simulink model "bh_smd_MAIN_HELLO_ORIG"  (R2018b)
settings: Solver=ode45  StartTime=0.0  StopTime=10.0  RelTol=1e-7
undefined symbols (not defined in the file or in its folder): c, k, m, x_init, xdot_init
settings Model: Creator=bhorton  LastModifiedBy=student
settings DebuggingCC: LibraryContextMissingDiagnostic=none
settings SFSimCC: SimUseLocalCustomCode=off
settings RTWCC: RTWUseLocalCustomCode=off
settings CodeAppCC: StateflowObjectComments=on

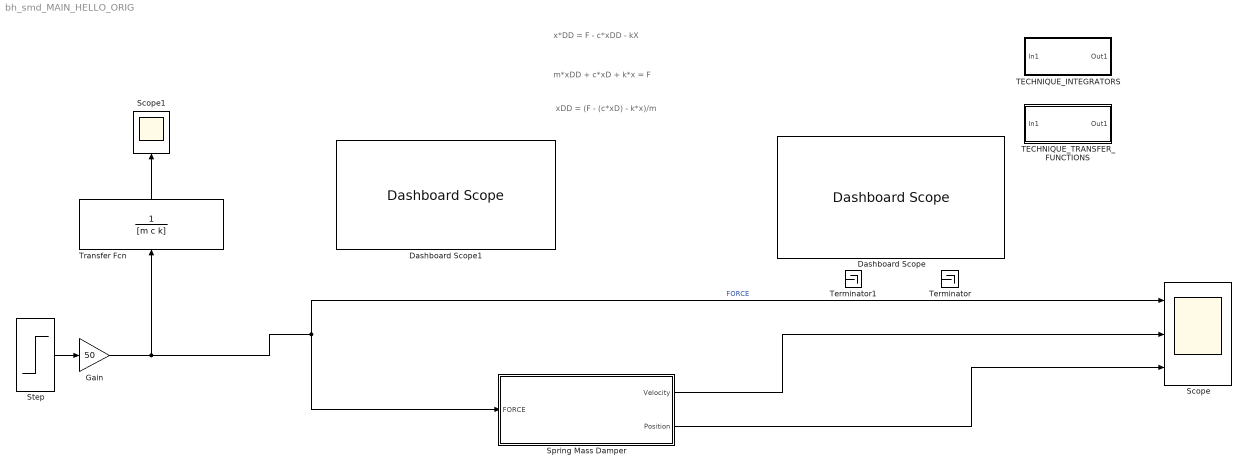
== system bh_smd_MAIN_HELLO_ORIG ==
  note: x*DD = F - c*xDD - kX
  note: xDD = (F - (c*xD) - k*x)/m
  note: m*xDD + c*xD + k*x = F
  Dashboard Scope : DashboardScope  WebBlockId=96
  Dashboard Scope1 : DashboardScope  WebBlockId=97
  Gain : Gain  Gain=50
  Scope : Scope  NumInputPorts=3
  Scope1 : Scope
  Spring Mass Damper : Subsystem
  Step : Step  Time=5  SampleTime=0
  TECHNIQUE_INTEGRATORS : Subsystem
  TECHNIQUE_TRANSFER_FUNCTIONS : Subsystem
  Terminator : Terminator
  Terminator1 : Terminator
  Transfer Fcn : TransferFcn  Denominator=[m c k]
  wires:
  Step/1 -> Gain/1
  Gain/1 -> Spring Mass Damper/1(FORCE), Scope/1, Transfer Fcn/1  "FORCE"
  Spring Mass Damper/1(Velocity) -> Scope/2
  Spring Mass Damper/2(Position) -> Scope/3
  Transfer Fcn/1 -> Scope1/1

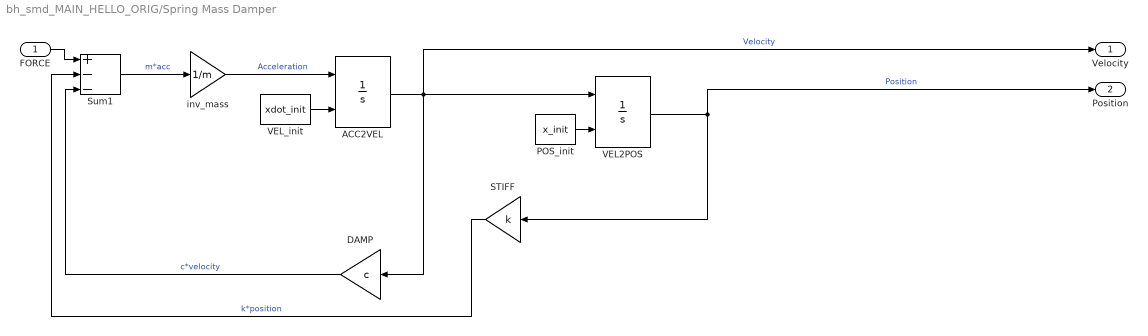
== system bh_smd_MAIN_HELLO_ORIG/Spring Mass Damper ==
  FORCE : Inport
  ACC2VEL : Integrator  InitialConditionSource=external
  "DAMP " : Gain  Gain=c
  POS_init : Constant  Value=x_init
  STIFF : Gain  Gain=k
  Sum1 : Sum  Inputs=+|-|-
  VEL2POS : Integrator  InitialConditionSource=external
  VEL_init : Constant  Value=xdot_init
  inv_mass : Gain  Gain=1/m
  Velocity : Outport
  Position : Outport  Port=2
  wires:
  Sum1/1 -> inv_mass/1  "m*acc"
  "DAMP "/1 -> Sum1/3  "c*velocity"
  VEL_init/1 -> ACC2VEL/2
  ACC2VEL/1 -> Velocity/1, "DAMP "/1, VEL2POS/1  "Velocity"
  POS_init/1 -> VEL2POS/2
  STIFF/1 -> Sum1/2  "k*position"
  inv_mass/1 -> ACC2VEL/1  "Acceleration"
  FORCE/1 -> Sum1/1
  VEL2POS/1 -> Position/1, STIFF/1  "Position"

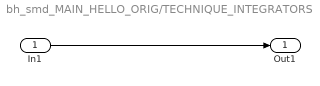
== system bh_smd_MAIN_HELLO_ORIG/TECHNIQUE_INTEGRATORS ==
  In1 : Inport
  Out1 : Outport
  wires:
  In1/1 -> Out1/1

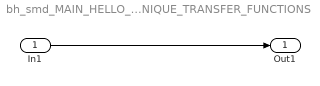
== system bh_smd_MAIN_HELLO_ORIG/TECHNIQUE_TRANSFER_FUNCTIONS ==
  In1 : Inport
  Out1 : Outport
  wires:
  In1/1 -> Out1/1
